simulink model "lab3_step4"  (R2019b)
settings: Solver=VariableStepAuto  StartTime=0.0  StopTime=stop_time  RelTol=1e-3
InitFcn:
  | %Read in the audio file
  | [input_wav_signal, Fs_in] = audioread('acoustic.wav');
  | % Fs_in = 11025 and we need to convert this to Fs = 48k
  | 
  | % Convert the Sampling rate to 48 kHz
  | signal = resample(input_wav_signal, 48000, 11025);
  | Fs = 48000; % This is out desired sample rate that we converted to
  | Ts = 1/Fs;    % and the associated sample period.
  | 
  | % Put signal into a timeseries format
  | timevals = [0:length(signal)-1]*Ts;
  | input_signal = timeseries(signal,timevals);
  | 
  | % Set the simulation stop time
  | stop_time = length(signal) * Ts; % set the simulation time the same length as the input signal
  | 
  | 
  | % Fixed-point precision we want the signal converted to.
  | W_bits = 32;
  | F_bits = 28;
  | 
  | max_reset_Nsamples = 1024*16 % should be a power of 2
  | max_reset_Nbits = ceil (log2 (max_reset_Nsamples));
StopFcn:
  | y_out = output_signal.Data(:);
  | plot(y_out)
  | soundsc(y_out,Fs)
undefined symbols (not defined in the file): magnitude
libraries: simulink x3, hdlsllib x1
settings Model: Creator=yassi  LastModifiedBy=yassi
settings DataIOCC: ReturnWorkspaceOutputs=off

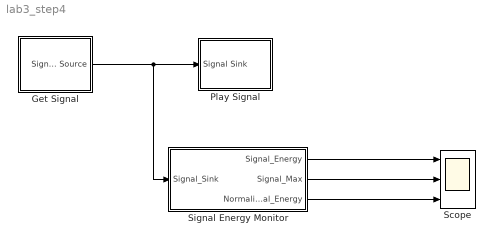
== system lab3_step4 ==
  Get Signal : Subsystem
  Play Signal : Subsystem
  Scope : Scope  NumInputPorts=3
  Signal Energy Monitor : Subsystem
  wires:
  Get Signal/1(Signal Source) -> Signal Energy Monitor/1(Signal_Sink), Play Signal/1(Signal Sink)
  Signal Energy Monitor/1(Signal_Energy) -> Scope/1
  Signal Energy Monitor/2(Signal_Max) -> Scope/2
  Signal Energy Monitor/3(Normalized_Signal_Energy) -> Scope/3

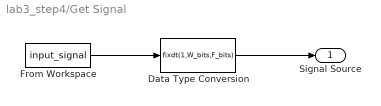
== system lab3_step4/Get Signal ==
  Data Type Conversion : DataTypeConversion  OutDataTypeStr=fixdt(1,W_bits,F_bits)
  From Workspace : FromWorkspace  VariableName=input_signal  SampleTime=Ts
  Signal Source : Outport
  wires:
  From Workspace/1 -> Data Type Conversion/1
  Data Type Conversion/1 -> Signal Source/1

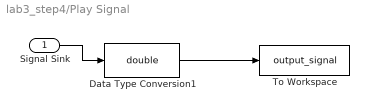
== system lab3_step4/Play Signal ==
  Signal Sink : Inport
  Data Type Conversion1 : DataTypeConversion  OutDataTypeStr=double
  To Workspace : ToWorkspace  VariableName=output_signal  SaveFormat=Timeseries  SampleTime=-1
  wires:
  Data Type Conversion1/1 -> To Workspace/1
  Signal Sink/1 -> Data Type Conversion1/1

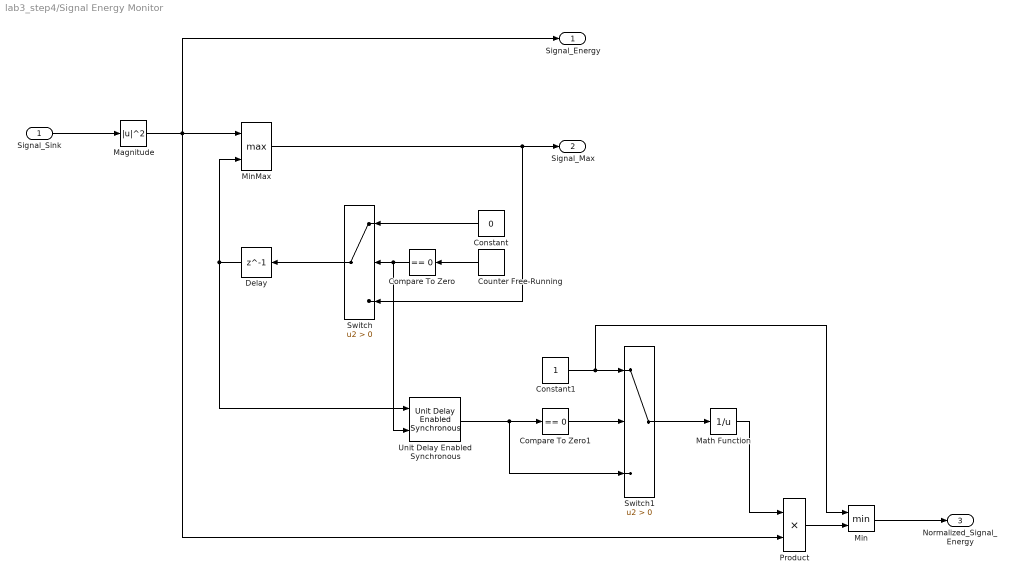
== system lab3_step4/Signal Energy Monitor ==
  Signal_Sink : Inport
  Compare To Zero : simulink/Logic and Bit Operations/Compare To Zero  relop===  OutDataTypeStr=boolean
  Compare To Zero1 : simulink/Logic and Bit Operations/Compare To Zero  relop===  OutDataTypeStr=boolean
  Constant : Constant  Value=0  OutDataTypeStr=fixdt(1,W_bits,F_bits)  SampleTime=Ts
  Constant1 : Constant  OutDataTypeStr=fixdt(1,W_bits,F_bits)  SampleTime=Ts
  Counter Free-Running : simulink/Sources/Counter Free-Running  NumBits=max_reset_Nbits  tsamp=Ts
  Delay : Delay  DelayLength=1
  Magnitude : Math  Operator=magnitude^2  RndMeth=Zero  SaturateOnIntegerOverflow=on
  Math Function : Math  Operator=reciprocal  SignedPower=off  OutDataTypeStr=fixdt(1,32,24)  SaturateOnIntegerOverflow=on
  Min : MinMax  Inputs=2
  MinMax : MinMax  Function=max  Inputs=2
  Product : Product  OutDataTypeStr=fixdt(1,32,28)
  Switch : Switch  Criteria=u2 > Threshold
  Switch1 : Switch  Criteria=u2 > Threshold
  Unit Delay Enabled Synchronous : hdlsllib/Discrete/Unit Delay Enabled Synchronous  InitialCondition=0.0  SampleTime=-1
      settings: SourceProductName=Simulink  SourceProductBaseCode=SL
  Signal_Energy : Outport
  Signal_Max : Outport  Port=2
  Normalized_Signal_Energy : Outport  Port=3
  wires:
  Magnitude/1 -> Product/2, Signal_Energy/1, MinMax/1
  MinMax/1 -> Switch/3, Signal_Max/1
  Delay/1 -> MinMax/2, Unit Delay Enabled Synchronous/1
  Signal_Sink/1 -> Magnitude/1
  Switch/1 -> Delay/1
  Constant/1 -> Switch/1
  Counter Free-Running/1 -> Compare To Zero/1
  Compare To Zero/1 -> Unit Delay Enabled Synchronous/2, Switch/2
  Math Function/1 -> Product/1
  Unit Delay Enabled Synchronous/1 -> Switch1/3, Compare To Zero1/1
  Constant1/1 -> Min/1, Switch1/1
  Compare To Zero1/1 -> Switch1/2
  Switch1/1 -> Math Function/1
  Product/1 -> Min/2
  Min/1 -> Normalized_Signal_Energy/1
